simulink model "carro_pendulo_TS_fuzzyM_2014"  (R2014b)
settings: Solver=ode3  StartTime=0.0  StopTime=inf  FixedStep=h  RelTol=1e-3
values from neighbouring files (symbols this model uses):
  g = 9.81    [LQR_Ganancias.m]
  h = 0.001    [LQR_Ganancias.m]
  I = 0.0260    (= 0.026)    [LQR_Ganancias.m]
  l = 0.641    [LQR_Ganancias.m]
  m = 0.23    [LQR_Ganancias.m]
  M = 0.57    [LQR_Ganancias.m]
undefined symbols (not defined in the file or in its folder): National_Instruments, PCI
libraries: rtwinlib x4, fuzblock x2
settings Model: SimulationMode=external  CovSFcnEnable=on  Creator=Jovani  LastModifiedBy=js231
settings DebuggingCC: UnderspecifiedInitializationDetection=Classic  MergeDetectMultiDrivingBlocksExec=none  FrameProcessingCompatibilityMsg=error  StateNameClashWarn=warning
settings HardwareCC: ProdBitPerPointer=64  ProdLargestAtomicFloat=Float  ProdIntDivRoundTo=Zero  ProdEndianess=LittleEndian  ProdHWDeviceType=Specified  TargetBitPerLong=64  TargetBitPerPointer=64  TargetIntDivRoundTo=Zero  TargetEndianess=LittleEndian  TargetWordSize=64  TargetHWDeviceType=Intel->x86-64
settings RTWCC: SystemTargetFile=rtwin.tlc  TemplateMakefile=rtwin.tmf  Description=Simulink Desktop Real-Time  RTWCompilerOptimization=On
settings CodeAppCC: MaxIdLength=95
settings RTWinTargetCC: TargetPreCompLibLocation=C:\Program Files\MATLAB\R2017b\toolbox\sldrt\lib\win64  GeneratePreprocessorConditionals=Use local settings  UseToolchainInfoCompliant=off  ExtModeMexFile=sldrtext

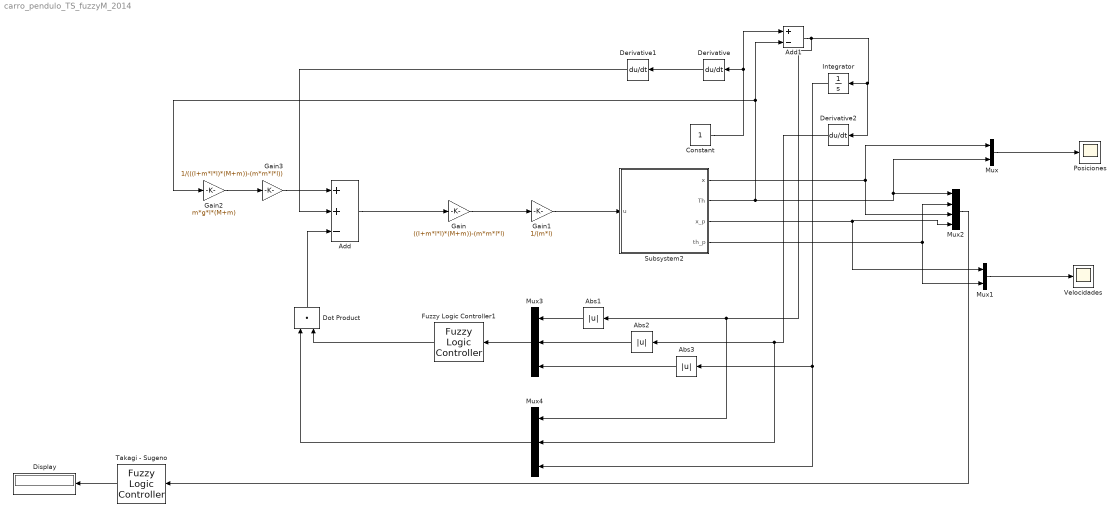
== system carro_pendulo_TS_fuzzyM_2014 ==
  Abs1 : Abs
  Abs2 : Abs
  Abs3 : Abs
  Add : Sum  Inputs=++-
  Add1 : Sum  Inputs=+-
  Constant : Constant
  Derivative : Derivative
  Derivative1 : Derivative
  Derivative2 : Derivative
  Display : Display
  Dot Product : DotProduct  InputSameDT=on  OutDataTypeStr=Inherit: Inherit via internal rule
  Fuzzy Logic Controller1 : fuzblock/Fuzzy Logic  Controller  FIS=M_carro_pendulo
  Gain : Gain  Gain=((I+m*l*l)*(M+m))-(m*m*l*l)
  Gain1 : Gain  Gain=1/(m*l)
  Gain2 : Gain  Gain=m*g*l*(M+m)
  Gain3 : Gain  Gain=1/(((I+m*l*l)*(M+m))-(m*m*l*l))
  Integrator : Integrator
  Mux : Mux  Inputs=2
  Mux1 : Mux  Inputs=2
  Mux2 : Mux
  Mux3 : Mux  Inputs=3
  Mux4 : Mux  Inputs=3
  "Posiciones " : Scope
      settings: TimeRange=auto  MaxDataPoints=5000  SaveToWorkspace=off  YMin=-10  YMax=10  SampleTime=-1
  Subsystem2 : Subsystem
  "Takagi - Sugeno " : fuzblock/Fuzzy Logic  Controller  FIS='TS carro pendulo.fis'
  "Velocidades " : Scope
      settings: TimeRange=auto  MaxDataPoints=5000  SaveToWorkspace=off  SaveName=ScopeData2  YMin=-10  YMax=10  SampleTime=-1
  wires:
  Mux2/1 -> "Takagi - Sugeno "/1
  Subsystem2/2(Th) -> Add1/2, Gain2/1, Mux/2, Mux2/1
  Subsystem2/4(th_p) -> Mux1/2, Mux2/2
  Subsystem2/1(x) -> Mux2/3, Mux/1
  Subsystem2/3(x_p) -> Mux1/1, Mux2/4
  Mux/1 -> "Posiciones "/1
  Mux1/1 -> "Velocidades "/1
  Gain1/1 -> Subsystem2/1(u)
  Gain/1 -> Gain1/1
  Add/1 -> Gain/1
  Gain2/1 -> Gain3/1
  Gain3/1 -> Add/1
  Constant/1 -> Derivative/1, Add1/1
  Derivative/1 -> Derivative1/1
  Derivative1/1 -> Add/2
  Abs3/1 -> Mux3/3
  Abs1/1 -> Mux3/1
  Mux3/1 -> Fuzzy Logic Controller1/1
  Fuzzy Logic Controller1/1 -> Dot Product/2
  Derivative2/1 -> Mux4/2, Abs2/1
  Mux4/1 -> Dot Product/1
  Abs2/1 -> Mux3/2
  Integrator/1 -> Mux4/3, Abs3/1
  Dot Product/1 -> Add/3
  Add1/1 -> Mux4/1, Abs1/1, Derivative2/1, Integrator/1
  "Takagi - Sugeno "/1 -> Display/1

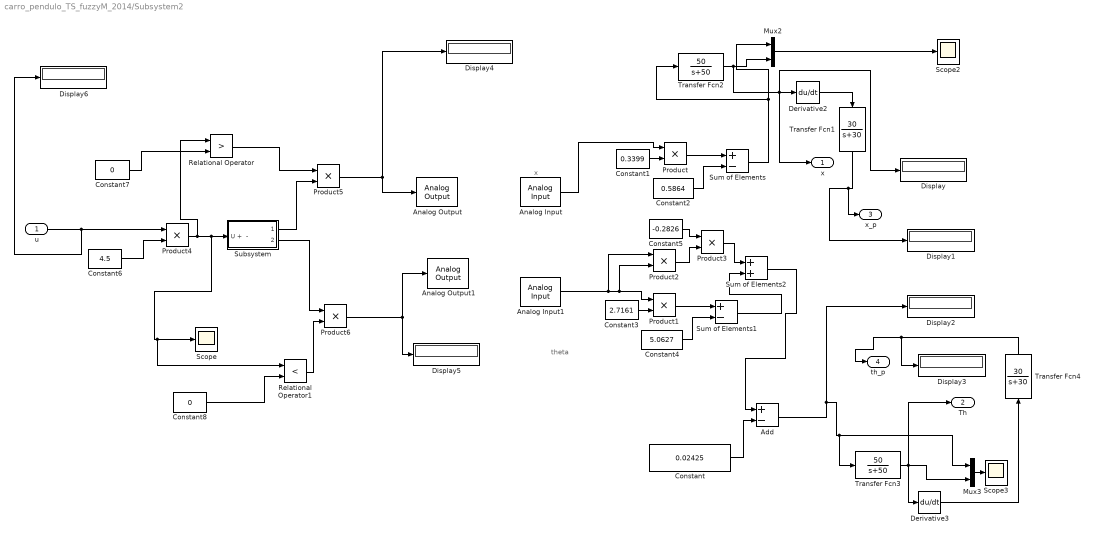
== system carro_pendulo_TS_fuzzyM_2014/Subsystem2 ==
  note: x
  note: theta
  u : Inport
  Add : Sum  Inputs=+-
  Analog Input : rtwinlib/Analog Input  SampleTime=h  MaxMissedTicks=10  ShowMissedTicks=off  YieldWhenWaiting=off  DrvName=National_Instruments/PCI-6071E  DrvAddress=0  DrvOptions=[0 0 0 0 0 0]  Channels=1  RangeMode=1  VoltRange=10  DataType=1
      settings: AttributesFormatString=National Instruments\nPCI-6071E [0h]
  Analog Input1 : rtwinlib/Analog Input  SampleTime=h  MaxMissedTicks=10  ShowMissedTicks=off  YieldWhenWaiting=off  DrvName=National_Instruments/PCI-6071E  DrvAddress=0  DrvOptions=[0 0 0 0 0 0]  Channels=2  RangeMode=1  VoltRange=10  DataType=1
      settings: AttributesFormatString=National Instruments\nPCI-6071E [0h]
  Analog Output : rtwinlib/Analog Output  SampleTime=h  MaxMissedTicks=10  ShowMissedTicks=off  YieldWhenWaiting=off  DrvName=National_Instruments/PCI-6071E  DrvAddress=0  DrvOptions=[0 0 0 0 0 0]  Channels=1  RangeMode=1  VoltRange=1  InitialValue=[]  FinalValue=[]
      settings: AttributesFormatString=National Instruments\nPCI-6071E [0h]
  Analog Output1 : rtwinlib/Analog Output  SampleTime=h  MaxMissedTicks=10  ShowMissedTicks=off  YieldWhenWaiting=off  DrvName=National_Instruments/PCI-6071E  DrvAddress=0  DrvOptions=[0 0 0 0 0 0]  Channels=2  RangeMode=1  VoltRange=1  InitialValue=[]  FinalValue=[]
      settings: AttributesFormatString=National Instruments\nPCI-6071E [0h]
  Constant : Constant  Value=0.02425
  Constant1 : Constant  Value=0.3399
  Constant2 : Constant  Value=0.5864
  Constant3 : Constant  Value=2.7161
  Constant4 : Constant  Value=5.0627
  Constant5 : Constant  Value=-0.2826
  Constant6 : Constant  Value=4.5
  Constant7 : Constant  Value=0
  Constant8 : Constant  Value=0
  Derivative2 : Derivative
  Derivative3 : Derivative
  Display{,1..6} (7 alike) : Display
  Mux2 : Mux  Inputs=2
  Mux3 : Mux  Inputs=2
  Product{,1..6} (7 alike) : Product
  Relational Operator : RelationalOperator  Operator=>  OutDataTypeStr=boolean
  Relational Operator1 : RelationalOperator  Operator=<  OutDataTypeStr=boolean
  Scope : Scope
      settings: TimeRange=auto  LimitDataPoints=on  MaxDataPoints=5000  SaveToWorkspace=off  SaveName=ScopeData2  YMin=-10  YMax=10  SampleTime=-1
  Scope2 : Scope
      settings: TimeRange=auto  MaxDataPoints=5000  SaveToWorkspace=off  SaveName=ScopeData3  YMin=-0.00775  YMax=-0.00575  SampleTime=-1
  Scope3 : Scope
      settings: TimeRange=auto  MaxDataPoints=5000  SaveToWorkspace=off  SaveName=ScopeData5  YMin=-0.4  YMax=0.45  SampleTime=-1
  Subsystem : Subsystem
  Sum of Elements : Sum  Inputs=+-
  Sum of Elements1 : Sum  Inputs=+-
  Sum of Elements2 : Sum
  Transfer Fcn1 : TransferFcn  Numerator=[30]  Denominator=[1 30]
  Transfer Fcn2 : TransferFcn  Numerator=[50]  Denominator=[1 50]
  Transfer Fcn3 : TransferFcn  Numerator=[50]  Denominator=[1 50]
  Transfer Fcn4 : TransferFcn  Numerator=[30]  Denominator=[1 30]
  x : Outport
  Th : Outport  Port=2
  x_p : Outport  Port=3
  th_p : Outport  Port=4
  wires:
  Transfer Fcn4/1 -> th_p/1, Display3/1
  Transfer Fcn1/1 -> x_p/1, Display1/1
  Transfer Fcn3/1 -> Mux3/2, Derivative3/1, Th/1
  Mux3/1 -> Scope3/1
  Transfer Fcn2/1 -> Mux2/2, Derivative2/1, Display/1, x/1
  Mux2/1 -> Scope2/1
  Derivative3/1 -> Transfer Fcn4/1
  Derivative2/1 -> Transfer Fcn1/1
  Subsystem/2(neg ++) -> Product6/1
  Subsystem/1(pos ++) -> Product5/2
  Constant/1 -> Add/2
  Sum of Elements2/1 -> Add/1
  Relational Operator/1 -> Product5/1
  Product6/1 -> Analog Output1/1, Display5/1
  Relational Operator1/1 -> Product6/2
  Constant8/1 -> Relational Operator1/2
  Product5/1 -> Display4/1, Analog Output/1
  Constant7/1 -> Relational Operator/2
  Product4/1 -> Subsystem/1(U +  -), Scope/1, Relational Operator1/1, Relational Operator/1
  Constant6/1 -> Product4/2
  u/1 -> Product4/1, Display6/1
  Sum of Elements1/1 -> Sum of Elements2/2
  Product3/1 -> Sum of Elements2/1
  Product2/1 -> Product3/2
  Constant5/1 -> Product3/1
  Constant4/1 -> Sum of Elements1/2
  Constant3/1 -> Product1/2
  Product1/1 -> Sum of Elements1/1
  Sum of Elements/1 -> Transfer Fcn2/1, Mux2/1
  Constant2/1 -> Sum of Elements/2
  Constant1/1 -> Product/2
  Product/1 -> Sum of Elements/1
  Analog Input/1 -> Product/1
  Analog Input1/1 -> Product1/1, Product2/2, Product2/1
  Add/1 -> Mux3/1, Transfer Fcn3/1, Display2/1

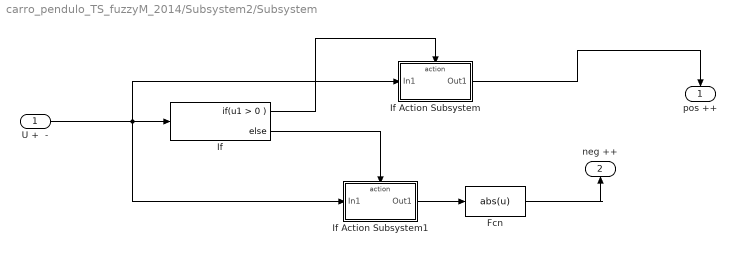
== system carro_pendulo_TS_fuzzyM_2014/Subsystem2/Subsystem ==
  U +  - : Inport
  Fcn : Fcn  Expr=abs(u)
  If : If  IfExpression=u1 > 0
  If Action Subsystem : Subsystem  TreatAsAtomicUnit=on
  If Action Subsystem1 : Subsystem  TreatAsAtomicUnit=on
  pos ++ : Outport
  neg ++ : Outport  Port=2
  wires:
  Fcn/1 -> neg ++/1
  If Action Subsystem1/1(Out1) -> Fcn/1
  If Action Subsystem/1(Out1) -> pos ++/1
  If/2 -> If Action Subsystem1/Action
  U +  -/1 -> If/1, If Action Subsystem/1(In1), If Action Subsystem1/1(In1)
  If/1 -> If Action Subsystem/Action

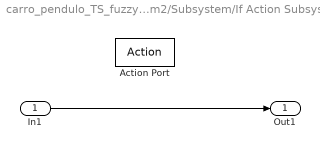
== system carro_pendulo_TS_fuzzyM_2014/Subsystem2/Subsystem/If Action Subsystem ==
  In1 : Inport
  Action Port : ActionPort  ActionType=then
  Out1 : Outport
  wires:
  In1/1 -> Out1/1

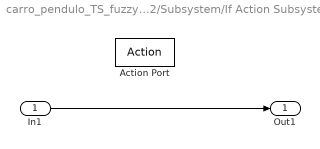
== system carro_pendulo_TS_fuzzyM_2014/Subsystem2/Subsystem/If Action Subsystem1 ==
  In1 : Inport
  Action Port : ActionPort  ActionType=else
  Out1 : Outport
  wires:
  In1/1 -> Out1/1
